simulink model "PC_CONTROL_STATION"  (R2023b)
settings: Solver=FixedStepAuto  StartTime=0.0  StopTime=inf  RelTol=1e-3  EnableMultiTasking=on
InitFcn:
  | if RUN_MODE~=5
  |     % clear rpi;
  |     rpi = raspberrypi(CAR_IP, 'pi', 'LabControl');
  |     stopModel(rpi,'CAR_CONTROL_SYSTEM')
  |     while isModelRunning(rpi,'CAR_CONTROL_SYSTEM')
  |          stopModel(rpi,'CAR_CONTROL_SYSTEM')
  |     end
  |     runModel(rpi,'CAR_CONTROL_SYSTEM')
  |      while isModelRunning(rpi,'CAR_CONTROL_SYSTEM')==false
  |          runModel(rpi,'CAR_CONTROL_SYSTEM')
  |      end
  |      % clear rpi;
  | end
StopFcn:
  | if RUN_MODE~=5
  |    clear rpi;
  |    rpi = raspberrypi(CAR_IP, 'pi', 'LabControl');
  |    stopModel(rpi,'CAR_CONTROL_SYSTEM')
  |    while isModelRunning(rpi,'CAR_CONTROL_SYSTEM')
  |    end
  |    clear rpi;
  | end
model workspace (MAT data in the model file):
  SL_ROS_VariableLengthArrays_MaxSizes : object (value not decoded)
values from neighbouring files (symbols this model uses):
  data = theClient.GetLastFrameOfData()    [FuncMotive.m]
undefined symbols (not defined in the file or in its folder): CONTROL, CONTROL_INI, data_SL_Info, MD25, MSG, SAMPLING_TIME, Standard_Devices, SYSID_INPUT, TCP_Protocol, UDP_Protocol
libraries: simulink x51, sldrtlib x46, dspsigattribs x7, ros2lib x3, ctrlSharedLib x2, aerolibanimutils x1
(part 3 of 8)

== system PC_CONTROL_STATION/HARDWARE/RT_MONITORING/TCP 106/MSG_TX  ==
  Enable : EnablePort
  Data Store Read1 : DataStoreRead  DataStoreName=MSG  SampleTime=CONTROL_INI.PARAM.COMM_SAMPLING_TIME  DataStoreElements=MSG.TX_BUFFER(:,1)  IndexOptions=Index vector (dialog)  Indices=1  OutputSizes=1
  Packet Output : sldrtlib/Packet Output  SampleTime=CONTROL_INI.PARAM.COMM_SAMPLING_TIME  MaxMissedTicks=50  ShowMissedTicks=off  YieldWhenWaiting=off  DrvName=Standard_Devices/TCP_Protocol  DrvAddress=27000  DrvOptions=[0 27001 49 57 50 46 49 54 56 46 48 46 49 48 54 0 0 0 0 0 0 0 0 0 0 0 0 0 0 0 0 0 0 0 0 0 0 0 0 0 0 0 0 0 0 0 0 0 0 0 0 0 0 0 0 0 0 0 0 0 0 0 0 0 0 0 0 0 0 0 0 0 0 0 0 0 0 0 0 0 0 0 0 0 0 0 0 0 0 0 0 0 0 0 0 0 0 0 0 0 0 0 0 0 0 0 0 0 0 0 0 0 0 0 0 0 0 0 0 0 0 0 0 0 0 0 0 0 0 0 0 0 0 0 0 0 0 0 0 0 0 0 0 0 0 0 0 0 0 0 0 0 0 0 0 0 0 0 0 0 0 0 0 0 0 0 0 0 0 0 0 0 0 0 0 0 0 0 0 0 0 0 0 0 0 0 0 0 0 0 0 0 0 0 0 0 0 0 0 0 0 0 0 0 0 0 0 0 0 0 0 0 0 0 0 0 0 0 0 0 0 0 0 0 0 0 0 0 0 0 0 0 0 0 0 0 0 0 0 0 0 0 0 0 0 0 0 0 0 0 0 0 0 0 0 0]  PacketSize=1400  DataTypes={'1400*uint8'}  ShowReady=off  ShowError=off  PacketID=1  ByteOrder=2  InitialValue=[]  FinalValue=[]
      settings: AttributesFormatString=TCP Protocol [27000]
  wires:
  Data Store Read1/1 -> Packet Output/1

== system PC_CONTROL_STATION/HARDWARE/RT_MONITORING/TCP 107/MSG_RX ==
  Bus Assignment : BusAssignment  AssignedSignals=RX_BUFFER
  Data Store Read : DataStoreRead  DataStoreName=MSG  IndexOptions=Index vector (dialog)  Indices=1  OutputSizes=1
  Data Store Write1 : DataStoreWrite  DataStoreName=MSG  IndexOptions=Index vector (dialog)  Indices=1  OutputSizes=1
  Packet Input : sldrtlib/Packet Input  SampleTime=CONTROL_INI.PARAM.COMM_SAMPLING_TIME  MaxMissedTicks=50  ShowMissedTicks=off  YieldWhenWaiting=off  DrvName=Standard_Devices/TCP_Protocol  DrvAddress=27001  DrvOptions=[0 27000 49 57 50 46 49 54 56 46 48 46 49 48 55 0 0 0 0 0 0 0 0 0 0 0 0 0 0 0 0 0 0 0 0 0 0 0 0 0 0 0 0 0 0 0 0 0 0 0 0 0 0 0 0 0 0 0 0 0 0 0 0 0 0 0 0 0 0 0 0 0 0 0 0 0 0 0 0 0 0 0 0 0 0 0 0 0 0 0 0 0 0 0 0 0 0 0 0 0 0 0 0 0 0 0 0 0 0 0 0 0 0 0 0 0 0 0 0 0 0 0 0 0 0 0 0 0 0 0 0 0 0 0 0 0 0 0 0 0 0 0 0 0 0 0 0 0 0 0 0 0 0 0 0 0 0 0 0 0 0 0 0 0 0 0 0 0 0 0 0 0 0 0 0 0 0 0 0 0 0 0 0 0 0 0 0 0 0 0 0 0 0 0 0 0 0 0 0 0 0 0 0 0 0 0 0 0 0 0 0 0 0 0 0 0 0 0 0 0 0 0 0 0 0 0 0 0 0 0 0 0 0 0 0 0 0 0 0 0 0 0 0 0 0 0 0 0 0 0 0 0 0 0 0 0]  PacketSize=1400  DataTypes={'1400*uint8'}  ShowReady=off  ShowError=off  PacketID=1  ByteOrder=2  ShowTimestamp=off
      settings: AttributesFormatString=TCP Protocol [27001]
  wires:
  Bus Assignment/1 -> Data Store Write1/1
  Data Store Read/1 -> Bus Assignment/1
  Packet Input/1 -> Bus Assignment/2

== system PC_CONTROL_STATION/HARDWARE/RT_MONITORING/TCP 107/MSG_TX  ==
  Enable : EnablePort
  Data Store Read1 : DataStoreRead  DataStoreName=MSG  SampleTime=CONTROL_INI.PARAM.COMM_SAMPLING_TIME  DataStoreElements=MSG.TX_BUFFER(:,1)  IndexOptions=Index vector (dialog)  Indices=1  OutputSizes=1
  Packet Output : sldrtlib/Packet Output  SampleTime=CONTROL_INI.PARAM.COMM_SAMPLING_TIME  MaxMissedTicks=50  ShowMissedTicks=off  YieldWhenWaiting=off  DrvName=Standard_Devices/TCP_Protocol  DrvAddress=27000  DrvOptions=[0 27001 49 57 50 46 49 54 56 46 48 46 49 48 55 0 0 0 0 0 0 0 0 0 0 0 0 0 0 0 0 0 0 0 0 0 0 0 0 0 0 0 0 0 0 0 0 0 0 0 0 0 0 0 0 0 0 0 0 0 0 0 0 0 0 0 0 0 0 0 0 0 0 0 0 0 0 0 0 0 0 0 0 0 0 0 0 0 0 0 0 0 0 0 0 0 0 0 0 0 0 0 0 0 0 0 0 0 0 0 0 0 0 0 0 0 0 0 0 0 0 0 0 0 0 0 0 0 0 0 0 0 0 0 0 0 0 0 0 0 0 0 0 0 0 0 0 0 0 0 0 0 0 0 0 0 0 0 0 0 0 0 0 0 0 0 0 0 0 0 0 0 0 0 0 0 0 0 0 0 0 0 0 0 0 0 0 0 0 0 0 0 0 0 0 0 0 0 0 0 0 0 0 0 0 0 0 0 0 0 0 0 0 0 0 0 0 0 0 0 0 0 0 0 0 0 0 0 0 0 0 0 0 0 0 0 0 0 0 0 0 0 0 0 0 0 0 0 0 0 0 0 0 0 0 0]  PacketSize=1400  DataTypes={'1400*uint8'}  ShowReady=off  ShowError=off  PacketID=1  ByteOrder=2  InitialValue=[]  FinalValue=[]
      settings: AttributesFormatString=TCP Protocol [27000]
  wires:
  Data Store Read1/1 -> Packet Output/1

== system PC_CONTROL_STATION/HARDWARE/RT_MONITORING/TCP 108/MSG_RX ==
  Bus Assignment : BusAssignment  AssignedSignals=RX_BUFFER
  Data Store Read : DataStoreRead  DataStoreName=MSG  IndexOptions=Index vector (dialog)  Indices=1  OutputSizes=1
  Data Store Write1 : DataStoreWrite  DataStoreName=MSG  IndexOptions=Index vector (dialog)  Indices=1  OutputSizes=1
  Packet Input : sldrtlib/Packet Input  SampleTime=CONTROL_INI.PARAM.COMM_SAMPLING_TIME  MaxMissedTicks=50  ShowMissedTicks=off  YieldWhenWaiting=off  DrvName=Standard_Devices/TCP_Protocol  DrvAddress=27001  DrvOptions=[0 27000 49 57 50 46 49 54 56 46 48 46 49 48 56 0 0 0 0 0 0 0 0 0 0 0 0 0 0 0 0 0 0 0 0 0 0 0 0 0 0 0 0 0 0 0 0 0 0 0 0 0 0 0 0 0 0 0 0 0 0 0 0 0 0 0 0 0 0 0 0 0 0 0 0 0 0 0 0 0 0 0 0 0 0 0 0 0 0 0 0 0 0 0 0 0 0 0 0 0 0 0 0 0 0 0 0 0 0 0 0 0 0 0 0 0 0 0 0 0 0 0 0 0 0 0 0 0 0 0 0 0 0 0 0 0 0 0 0 0 0 0 0 0 0 0 0 0 0 0 0 0 0 0 0 0 0 0 0 0 0 0 0 0 0 0 0 0 0 0 0 0 0 0 0 0 0 0 0 0 0 0 0 0 0 0 0 0 0 0 0 0 0 0 0 0 0 0 0 0 0 0 0 0 0 0 0 0 0 0 0 0 0 0 0 0 0 0 0 0 0 0 0 0 0 0 0 0 0 0 0 0 0 0 0 0 0 0 0 0 0 0 0 0 0 0 0 0 0 0 0 0 0 0 0 0]  PacketSize=1400  DataTypes={'1400*uint8'}  ShowReady=off  ShowError=off  PacketID=1  ByteOrder=2  ShowTimestamp=off
      settings: AttributesFormatString=TCP Protocol [27001]
  wires:
  Bus Assignment/1 -> Data Store Write1/1
  Data Store Read/1 -> Bus Assignment/1
  Packet Input/1 -> Bus Assignment/2

== system PC_CONTROL_STATION/HARDWARE/RT_MONITORING/TCP 108/MSG_TX  ==
  Enable : EnablePort
  Data Store Read1 : DataStoreRead  DataStoreName=MSG  SampleTime=CONTROL_INI.PARAM.COMM_SAMPLING_TIME  DataStoreElements=MSG.TX_BUFFER(:,1)  IndexOptions=Index vector (dialog)  Indices=1  OutputSizes=1
  Packet Output : sldrtlib/Packet Output  SampleTime=CONTROL_INI.PARAM.COMM_SAMPLING_TIME  MaxMissedTicks=50  ShowMissedTicks=off  YieldWhenWaiting=off  DrvName=Standard_Devices/TCP_Protocol  DrvAddress=27000  DrvOptions=[0 27001 49 57 50 46 49 54 56 46 48 46 49 48 56 0 0 0 0 0 0 0 0 0 0 0 0 0 0 0 0 0 0 0 0 0 0 0 0 0 0 0 0 0 0 0 0 0 0 0 0 0 0 0 0 0 0 0 0 0 0 0 0 0 0 0 0 0 0 0 0 0 0 0 0 0 0 0 0 0 0 0 0 0 0 0 0 0 0 0 0 0 0 0 0 0 0 0 0 0 0 0 0 0 0 0 0 0 0 0 0 0 0 0 0 0 0 0 0 0 0 0 0 0 0 0 0 0 0 0 0 0 0 0 0 0 0 0 0 0 0 0 0 0 0 0 0 0 0 0 0 0 0 0 0 0 0 0 0 0 0 0 0 0 0 0 0 0 0 0 0 0 0 0 0 0 0 0 0 0 0 0 0 0 0 0 0 0 0 0 0 0 0 0 0 0 0 0 0 0 0 0 0 0 0 0 0 0 0 0 0 0 0 0 0 0 0 0 0 0 0 0 0 0 0 0 0 0 0 0 0 0 0 0 0 0 0 0 0 0 0 0 0 0 0 0 0 0 0 0 0 0 0 0 0 0]  PacketSize=1400  DataTypes={'1400*uint8'}  ShowReady=off  ShowError=off  PacketID=1  ByteOrder=2  InitialValue=[]  FinalValue=[]
      settings: AttributesFormatString=TCP Protocol [27000]
  wires:
  Data Store Read1/1 -> Packet Output/1

== system PC_CONTROL_STATION/HARDWARE/RT_MONITORING/TCP 109/MSG_RX ==
  Bus Assignment : BusAssignment  AssignedSignals=RX_BUFFER
  Data Store Read : DataStoreRead  DataStoreName=MSG  IndexOptions=Index vector (dialog)  Indices=1  OutputSizes=1
  Data Store Write1 : DataStoreWrite  DataStoreName=MSG  IndexOptions=Index vector (dialog)  Indices=1  OutputSizes=1
  Packet Input : sldrtlib/Packet Input  SampleTime=CONTROL_INI.PARAM.COMM_SAMPLING_TIME  MaxMissedTicks=50  ShowMissedTicks=off  YieldWhenWaiting=off  DrvName=Standard_Devices/TCP_Protocol  DrvAddress=27001  DrvOptions=[0 27000 49 57 50 46 49 54 56 46 48 46 49 48 57 0 0 0 0 0 0 0 0 0 0 0 0 0 0 0 0 0 0 0 0 0 0 0 0 0 0 0 0 0 0 0 0 0 0 0 0 0 0 0 0 0 0 0 0 0 0 0 0 0 0 0 0 0 0 0 0 0 0 0 0 0 0 0 0 0 0 0 0 0 0 0 0 0 0 0 0 0 0 0 0 0 0 0 0 0 0 0 0 0 0 0 0 0 0 0 0 0 0 0 0 0 0 0 0 0 0 0 0 0 0 0 0 0 0 0 0 0 0 0 0 0 0 0 0 0 0 0 0 0 0 0 0 0 0 0 0 0 0 0 0 0 0 0 0 0 0 0 0 0 0 0 0 0 0 0 0 0 0 0 0 0 0 0 0 0 0 0 0 0 0 0 0 0 0 0 0 0 0 0 0 0 0 0 0 0 0 0 0 0 0 0 0 0 0 0 0 0 0 0 0 0 0 0 0 0 0 0 0 0 0 0 0 0 0 0 0 0 0 0 0 0 0 0 0 0 0 0 0 0 0 0 0 0 0 0 0 0 0 0 0 0]  PacketSize=1400  DataTypes={'1400*uint8'}  ShowReady=off  ShowError=off  PacketID=1  ByteOrder=2  ShowTimestamp=off
      settings: AttributesFormatString=TCP Protocol [27001]
  wires:
  Bus Assignment/1 -> Data Store Write1/1
  Data Store Read/1 -> Bus Assignment/1
  Packet Input/1 -> Bus Assignment/2

== system PC_CONTROL_STATION/HARDWARE/RT_MONITORING/TCP 109/MSG_TX  ==
  Enable : EnablePort
  Data Store Read1 : DataStoreRead  DataStoreName=MSG  SampleTime=CONTROL_INI.PARAM.COMM_SAMPLING_TIME  DataStoreElements=MSG.TX_BUFFER(:,1)  IndexOptions=Index vector (dialog)  Indices=1  OutputSizes=1
  Packet Output : sldrtlib/Packet Output  SampleTime=CONTROL_INI.PARAM.COMM_SAMPLING_TIME  MaxMissedTicks=50  ShowMissedTicks=off  YieldWhenWaiting=off  DrvName=Standard_Devices/TCP_Protocol  DrvAddress=27000  DrvOptions=[0 27001 49 57 50 46 49 54 56 46 48 46 49 48 57 0 0 0 0 0 0 0 0 0 0 0 0 0 0 0 0 0 0 0 0 0 0 0 0 0 0 0 0 0 0 0 0 0 0 0 0 0 0 0 0 0 0 0 0 0 0 0 0 0 0 0 0 0 0 0 0 0 0 0 0 0 0 0 0 0 0 0 0 0 0 0 0 0 0 0 0 0 0 0 0 0 0 0 0 0 0 0 0 0 0 0 0 0 0 0 0 0 0 0 0 0 0 0 0 0 0 0 0 0 0 0 0 0 0 0 0 0 0 0 0 0 0 0 0 0 0 0 0 0 0 0 0 0 0 0 0 0 0 0 0 0 0 0 0 0 0 0 0 0 0 0 0 0 0 0 0 0 0 0 0 0 0 0 0 0 0 0 0 0 0 0 0 0 0 0 0 0 0 0 0 0 0 0 0 0 0 0 0 0 0 0 0 0 0 0 0 0 0 0 0 0 0 0 0 0 0 0 0 0 0 0 0 0 0 0 0 0 0 0 0 0 0 0 0 0 0 0 0 0 0 0 0 0 0 0 0 0 0 0 0 0]  PacketSize=1400  DataTypes={'1400*uint8'}  ShowReady=off  ShowError=off  PacketID=1  ByteOrder=2  InitialValue=[]  FinalValue=[]
      settings: AttributesFormatString=TCP Protocol [27000]
  wires:
  Data Store Read1/1 -> Packet Output/1

== system PC_CONTROL_STATION/HARDWARE/RT_MONITORING/TCP 110/MSG_RX ==
  Bus Assignment : BusAssignment  AssignedSignals=RX_BUFFER
  Data Store Read : DataStoreRead  DataStoreName=MSG  IndexOptions=Index vector (dialog)  Indices=1  OutputSizes=1
  Data Store Write1 : DataStoreWrite  DataStoreName=MSG  IndexOptions=Index vector (dialog)  Indices=1  OutputSizes=1
  Packet Input : sldrtlib/Packet Input  SampleTime=CONTROL_INI.PARAM.COMM_SAMPLING_TIME  MaxMissedTicks=50  ShowMissedTicks=off  YieldWhenWaiting=off  DrvName=Standard_Devices/TCP_Protocol  DrvAddress=27001  DrvOptions=[0 27000 49 57 50 46 49 54 56 46 48 46 49 49 48 0 0 0 0 0 0 0 0 0 0 0 0 0 0 0 0 0 0 0 0 0 0 0 0 0 0 0 0 0 0 0 0 0 0 0 0 0 0 0 0 0 0 0 0 0 0 0 0 0 0 0 0 0 0 0 0 0 0 0 0 0 0 0 0 0 0 0 0 0 0 0 0 0 0 0 0 0 0 0 0 0 0 0 0 0 0 0 0 0 0 0 0 0 0 0 0 0 0 0 0 0 0 0 0 0 0 0 0 0 0 0 0 0 0 0 0 0 0 0 0 0 0 0 0 0 0 0 0 0 0 0 0 0 0 0 0 0 0 0 0 0 0 0 0 0 0 0 0 0 0 0 0 0 0 0 0 0 0 0 0 0 0 0 0 0 0 0 0 0 0 0 0 0 0 0 0 0 0 0 0 0 0 0 0 0 0 0 0 0 0 0 0 0 0 0 0 0 0 0 0 0 0 0 0 0 0 0 0 0 0 0 0 0 0 0 0 0 0 0 0 0 0 0 0 0 0 0 0 0 0 0 0 0 0 0 0 0 0 0 0 0]  PacketSize=1400  DataTypes={'1400*uint8'}  ShowReady=off  ShowError=off  PacketID=1  ByteOrder=2  ShowTimestamp=off
      settings: AttributesFormatString=TCP Protocol [27001]
  wires:
  Bus Assignment/1 -> Data Store Write1/1
  Data Store Read/1 -> Bus Assignment/1
  Packet Input/1 -> Bus Assignment/2

== system PC_CONTROL_STATION/HARDWARE/RT_MONITORING/TCP 110/MSG_TX  ==
  Enable : EnablePort
  Data Store Read1 : DataStoreRead  DataStoreName=MSG  SampleTime=CONTROL_INI.PARAM.COMM_SAMPLING_TIME  DataStoreElements=MSG.TX_BUFFER(:,1)  IndexOptions=Index vector (dialog)  Indices=1  OutputSizes=1
  Packet Output : sldrtlib/Packet Output  SampleTime=CONTROL_INI.PARAM.COMM_SAMPLING_TIME  MaxMissedTicks=50  ShowMissedTicks=off  YieldWhenWaiting=off  DrvName=Standard_Devices/TCP_Protocol  DrvAddress=27000  DrvOptions=[0 27001 49 57 50 46 49 54 56 46 48 46 49 49 48 0 0 0 0 0 0 0 0 0 0 0 0 0 0 0 0 0 0 0 0 0 0 0 0 0 0 0 0 0 0 0 0 0 0 0 0 0 0 0 0 0 0 0 0 0 0 0 0 0 0 0 0 0 0 0 0 0 0 0 0 0 0 0 0 0 0 0 0 0 0 0 0 0 0 0 0 0 0 0 0 0 0 0 0 0 0 0 0 0 0 0 0 0 0 0 0 0 0 0 0 0 0 0 0 0 0 0 0 0 0 0 0 0 0 0 0 0 0 0 0 0 0 0 0 0 0 0 0 0 0 0 0 0 0 0 0 0 0 0 0 0 0 0 0 0 0 0 0 0 0 0 0 0 0 0 0 0 0 0 0 0 0 0 0 0 0 0 0 0 0 0 0 0 0 0 0 0 0 0 0 0 0 0 0 0 0 0 0 0 0 0 0 0 0 0 0 0 0 0 0 0 0 0 0 0 0 0 0 0 0 0 0 0 0 0 0 0 0 0 0 0 0 0 0 0 0 0 0 0 0 0 0 0 0 0 0 0 0 0 0 0]  PacketSize=1400  DataTypes={'1400*uint8'}  ShowReady=off  ShowError=off  PacketID=1  ByteOrder=2  InitialValue=[]  FinalValue=[]
      settings: AttributesFormatString=TCP Protocol [27000]
  wires:
  Data Store Read1/1 -> Packet Output/1

== system PC_CONTROL_STATION/HARDWARE/RT_MONITORING/TCP 111/MSG_RX ==
  Bus Assignment : BusAssignment  AssignedSignals=RX_BUFFER
  Data Store Read : DataStoreRead  DataStoreName=MSG  IndexOptions=Index vector (dialog)  Indices=1  OutputSizes=1
  Data Store Write1 : DataStoreWrite  DataStoreName=MSG  IndexOptions=Index vector (dialog)  Indices=1  OutputSizes=1
  Packet Input : sldrtlib/Packet Input  SampleTime=CONTROL_INI.PARAM.COMM_SAMPLING_TIME  MaxMissedTicks=50  ShowMissedTicks=off  YieldWhenWaiting=off  DrvName=Standard_Devices/TCP_Protocol  DrvAddress=27001  DrvOptions=[0 27000 49 57 50 46 49 54 56 46 48 46 49 49 49 0 0 0 0 0 0 0 0 0 0 0 0 0 0 0 0 0 0 0 0 0 0 0 0 0 0 0 0 0 0 0 0 0 0 0 0 0 0 0 0 0 0 0 0 0 0 0 0 0 0 0 0 0 0 0 0 0 0 0 0 0 0 0 0 0 0 0 0 0 0 0 0 0 0 0 0 0 0 0 0 0 0 0 0 0 0 0 0 0 0 0 0 0 0 0 0 0 0 0 0 0 0 0 0 0 0 0 0 0 0 0 0 0 0 0 0 0 0 0 0 0 0 0 0 0 0 0 0 0 0 0 0 0 0 0 0 0 0 0 0 0 0 0 0 0 0 0 0 0 0 0 0 0 0 0 0 0 0 0 0 0 0 0 0 0 0 0 0 0 0 0 0 0 0 0 0 0 0 0 0 0 0 0 0 0 0 0 0 0 0 0 0 0 0 0 0 0 0 0 0 0 0 0 0 0 0 0 0 0 0 0 0 0 0 0 0 0 0 0 0 0 0 0 0 0 0 0 0 0 0 0 0 0 0 0 0 0 0 0 0 0]  PacketSize=1400  DataTypes={'1400*uint8'}  ShowReady=off  ShowError=off  PacketID=1  ByteOrder=2  ShowTimestamp=off
      settings: AttributesFormatString=TCP Protocol [27001]
  wires:
  Bus Assignment/1 -> Data Store Write1/1
  Data Store Read/1 -> Bus Assignment/1
  Packet Input/1 -> Bus Assignment/2

== system PC_CONTROL_STATION/HARDWARE/RT_MONITORING/TCP 111/MSG_TX  ==
  Enable : EnablePort
  Data Store Read1 : DataStoreRead  DataStoreName=MSG  SampleTime=CONTROL_INI.PARAM.COMM_SAMPLING_TIME  DataStoreElements=MSG.TX_BUFFER(:,1)  IndexOptions=Index vector (dialog)  Indices=1  OutputSizes=1
  Packet Output : sldrtlib/Packet Output  SampleTime=CONTROL_INI.PARAM.COMM_SAMPLING_TIME  MaxMissedTicks=50  ShowMissedTicks=off  YieldWhenWaiting=off  DrvName=Standard_Devices/TCP_Protocol  DrvAddress=27000  DrvOptions=[0 27001 49 57 50 46 49 54 56 46 48 46 49 49 49 0 0 0 0 0 0 0 0 0 0 0 0 0 0 0 0 0 0 0 0 0 0 0 0 0 0 0 0 0 0 0 0 0 0 0 0 0 0 0 0 0 0 0 0 0 0 0 0 0 0 0 0 0 0 0 0 0 0 0 0 0 0 0 0 0 0 0 0 0 0 0 0 0 0 0 0 0 0 0 0 0 0 0 0 0 0 0 0 0 0 0 0 0 0 0 0 0 0 0 0 0 0 0 0 0 0 0 0 0 0 0 0 0 0 0 0 0 0 0 0 0 0 0 0 0 0 0 0 0 0 0 0 0 0 0 0 0 0 0 0 0 0 0 0 0 0 0 0 0 0 0 0 0 0 0 0 0 0 0 0 0 0 0 0 0 0 0 0 0 0 0 0 0 0 0 0 0 0 0 0 0 0 0 0 0 0 0 0 0 0 0 0 0 0 0 0 0 0 0 0 0 0 0 0 0 0 0 0 0 0 0 0 0 0 0 0 0 0 0 0 0 0 0 0 0 0 0 0 0 0 0 0 0 0 0 0 0 0 0 0 0]  PacketSize=1400  DataTypes={'1400*uint8'}  ShowReady=off  ShowError=off  PacketID=1  ByteOrder=2  InitialValue=[]  FinalValue=[]
      settings: AttributesFormatString=TCP Protocol [27000]
  wires:
  Data Store Read1/1 -> Packet Output/1

== system PC_CONTROL_STATION/HARDWARE/RT_MONITORING/TCP 112/MSG_RX ==
  Bus Assignment : BusAssignment  AssignedSignals=RX_BUFFER
  Data Store Read : DataStoreRead  DataStoreName=MSG  IndexOptions=Index vector (dialog)  Indices=1  OutputSizes=1
  Data Store Write1 : DataStoreWrite  DataStoreName=MSG  IndexOptions=Index vector (dialog)  Indices=1  OutputSizes=1
  Packet Input : sldrtlib/Packet Input  SampleTime=CONTROL_INI.PARAM.COMM_SAMPLING_TIME  MaxMissedTicks=50  ShowMissedTicks=off  YieldWhenWaiting=off  DrvName=Standard_Devices/TCP_Protocol  DrvAddress=27001  DrvOptions=[0 27000 49 57 50 46 49 54 56 46 48 46 49 49 50 0 0 0 0 0 0 0 0 0 0 0 0 0 0 0 0 0 0 0 0 0 0 0 0 0 0 0 0 0 0 0 0 0 0 0 0 0 0 0 0 0 0 0 0 0 0 0 0 0 0 0 0 0 0 0 0 0 0 0 0 0 0 0 0 0 0 0 0 0 0 0 0 0 0 0 0 0 0 0 0 0 0 0 0 0 0 0 0 0 0 0 0 0 0 0 0 0 0 0 0 0 0 0 0 0 0 0 0 0 0 0 0 0 0 0 0 0 0 0 0 0 0 0 0 0 0 0 0 0 0 0 0 0 0 0 0 0 0 0 0 0 0 0 0 0 0 0 0 0 0 0 0 0 0 0 0 0 0 0 0 0 0 0 0 0 0 0 0 0 0 0 0 0 0 0 0 0 0 0 0 0 0 0 0 0 0 0 0 0 0 0 0 0 0 0 0 0 0 0 0 0 0 0 0 0 0 0 0 0 0 0 0 0 0 0 0 0 0 0 0 0 0 0 0 0 0 0 0 0 0 0 0 0 0 0 0 0 0 0 0 0]  PacketSize=1400  DataTypes={'1400*uint8'}  ShowReady=off  ShowError=off  PacketID=1  ByteOrder=2  ShowTimestamp=off
      settings: AttributesFormatString=TCP Protocol [27001]
  wires:
  Bus Assignment/1 -> Data Store Write1/1
  Data Store Read/1 -> Bus Assignment/1
  Packet Input/1 -> Bus Assignment/2

== system PC_CONTROL_STATION/HARDWARE/RT_MONITORING/TCP 112/MSG_TX  ==
  Enable : EnablePort
  Data Store Read1 : DataStoreRead  DataStoreName=MSG  SampleTime=CONTROL_INI.PARAM.COMM_SAMPLING_TIME  DataStoreElements=MSG.TX_BUFFER(:,1)  IndexOptions=Index vector (dialog)  Indices=1  OutputSizes=1
  Packet Output : sldrtlib/Packet Output  SampleTime=CONTROL_INI.PARAM.COMM_SAMPLING_TIME  MaxMissedTicks=50  ShowMissedTicks=off  YieldWhenWaiting=off  DrvName=Standard_Devices/TCP_Protocol  DrvAddress=27000  DrvOptions=[0 27001 49 57 50 46 49 54 56 46 48 46 49 49 50 0 0 0 0 0 0 0 0 0 0 0 0 0 0 0 0 0 0 0 0 0 0 0 0 0 0 0 0 0 0 0 0 0 0 0 0 0 0 0 0 0 0 0 0 0 0 0 0 0 0 0 0 0 0 0 0 0 0 0 0 0 0 0 0 0 0 0 0 0 0 0 0 0 0 0 0 0 0 0 0 0 0 0 0 0 0 0 0 0 0 0 0 0 0 0 0 0 0 0 0 0 0 0 0 0 0 0 0 0 0 0 0 0 0 0 0 0 0 0 0 0 0 0 0 0 0 0 0 0 0 0 0 0 0 0 0 0 0 0 0 0 0 0 0 0 0 0 0 0 0 0 0 0 0 0 0 0 0 0 0 0 0 0 0 0 0 0 0 0 0 0 0 0 0 0 0 0 0 0 0 0 0 0 0 0 0 0 0 0 0 0 0 0 0 0 0 0 0 0 0 0 0 0 0 0 0 0 0 0 0 0 0 0 0 0 0 0 0 0 0 0 0 0 0 0 0 0 0 0 0 0 0 0 0 0 0 0 0 0 0 0]  PacketSize=1400  DataTypes={'1400*uint8'}  ShowReady=off  ShowError=off  PacketID=1  ByteOrder=2  InitialValue=[]  FinalValue=[]
      settings: AttributesFormatString=TCP Protocol [27000]
  wires:
  Data Store Read1/1 -> Packet Output/1

== system PC_CONTROL_STATION/HARDWARE/RT_MONITORING/TCP 113/MSG_RX ==
  Bus Assignment : BusAssignment  AssignedSignals=RX_BUFFER
  Data Store Read : DataStoreRead  DataStoreName=MSG  IndexOptions=Index vector (dialog)  Indices=1  OutputSizes=1
  Data Store Write1 : DataStoreWrite  DataStoreName=MSG  IndexOptions=Index vector (dialog)  Indices=1  OutputSizes=1
  Packet Input : sldrtlib/Packet Input  SampleTime=CONTROL_INI.PARAM.COMM_SAMPLING_TIME  MaxMissedTicks=50  ShowMissedTicks=off  YieldWhenWaiting=off  DrvName=Standard_Devices/TCP_Protocol  DrvAddress=27001  DrvOptions=[0 27000 49 57 50 46 49 54 56 46 48 46 49 49 51 0 0 0 0 0 0 0 0 0 0 0 0 0 0 0 0 0 0 0 0 0 0 0 0 0 0 0 0 0 0 0 0 0 0 0 0 0 0 0 0 0 0 0 0 0 0 0 0 0 0 0 0 0 0 0 0 0 0 0 0 0 0 0 0 0 0 0 0 0 0 0 0 0 0 0 0 0 0 0 0 0 0 0 0 0 0 0 0 0 0 0 0 0 0 0 0 0 0 0 0 0 0 0 0 0 0 0 0 0 0 0 0 0 0 0 0 0 0 0 0 0 0 0 0 0 0 0 0 0 0 0 0 0 0 0 0 0 0 0 0 0 0 0 0 0 0 0 0 0 0 0 0 0 0 0 0 0 0 0 0 0 0 0 0 0 0 0 0 0 0 0 0 0 0 0 0 0 0 0 0 0 0 0 0 0 0 0 0 0 0 0 0 0 0 0 0 0 0 0 0 0 0 0 0 0 0 0 0 0 0 0 0 0 0 0 0 0 0 0 0 0 0 0 0 0 0 0 0 0 0 0 0 0 0 0 0 0 0 0 0 0]  PacketSize=1400  DataTypes={'1400*uint8'}  ShowReady=off  ShowError=off  PacketID=1  ByteOrder=2  ShowTimestamp=off
      settings: AttributesFormatString=TCP Protocol [27001]
  wires:
  Bus Assignment/1 -> Data Store Write1/1
  Data Store Read/1 -> Bus Assignment/1
  Packet Input/1 -> Bus Assignment/2

== system PC_CONTROL_STATION/HARDWARE/RT_MONITORING/TCP 113/MSG_TX  ==
  Enable : EnablePort
  Data Store Read1 : DataStoreRead  DataStoreName=MSG  SampleTime=CONTROL_INI.PARAM.COMM_SAMPLING_TIME  DataStoreElements=MSG.TX_BUFFER(:,1)  IndexOptions=Index vector (dialog)  Indices=1  OutputSizes=1
  Packet Output : sldrtlib/Packet Output  SampleTime=CONTROL_INI.PARAM.COMM_SAMPLING_TIME  MaxMissedTicks=50  ShowMissedTicks=off  YieldWhenWaiting=off  DrvName=Standard_Devices/TCP_Protocol  DrvAddress=27000  DrvOptions=[0 27001 49 57 50 46 49 54 56 46 48 46 49 49 51 0 0 0 0 0 0 0 0 0 0 0 0 0 0 0 0 0 0 0 0 0 0 0 0 0 0 0 0 0 0 0 0 0 0 0 0 0 0 0 0 0 0 0 0 0 0 0 0 0 0 0 0 0 0 0 0 0 0 0 0 0 0 0 0 0 0 0 0 0 0 0 0 0 0 0 0 0 0 0 0 0 0 0 0 0 0 0 0 0 0 0 0 0 0 0 0 0 0 0 0 0 0 0 0 0 0 0 0 0 0 0 0 0 0 0 0 0 0 0 0 0 0 0 0 0 0 0 0 0 0 0 0 0 0 0 0 0 0 0 0 0 0 0 0 0 0 0 0 0 0 0 0 0 0 0 0 0 0 0 0 0 0 0 0 0 0 0 0 0 0 0 0 0 0 0 0 0 0 0 0 0 0 0 0 0 0 0 0 0 0 0 0 0 0 0 0 0 0 0 0 0 0 0 0 0 0 0 0 0 0 0 0 0 0 0 0 0 0 0 0 0 0 0 0 0 0 0 0 0 0 0 0 0 0 0 0 0 0 0 0 0]  PacketSize=1400  DataTypes={'1400*uint8'}  ShowReady=off  ShowError=off  PacketID=1  ByteOrder=2  InitialValue=[]  FinalValue=[]
      settings: AttributesFormatString=TCP Protocol [27000]
  wires:
  Data Store Read1/1 -> Packet Output/1

== system PC_CONTROL_STATION/HARDWARE/RT_MONITORING/TCP 114/MSG_RX ==
  Bus Assignment : BusAssignment  AssignedSignals=RX_BUFFER
  Data Store Read : DataStoreRead  DataStoreName=MSG  IndexOptions=Index vector (dialog)  Indices=1  OutputSizes=1
  Data Store Write1 : DataStoreWrite  DataStoreName=MSG  IndexOptions=Index vector (dialog)  Indices=1  OutputSizes=1
  Packet Input : sldrtlib/Packet Input  SampleTime=CONTROL_INI.PARAM.COMM_SAMPLING_TIME  MaxMissedTicks=50  ShowMissedTicks=off  YieldWhenWaiting=off  DrvName=Standard_Devices/TCP_Protocol  DrvAddress=27001  DrvOptions=[0 27000 49 57 50 46 49 54 56 46 49 46 49 50 0 0 0 0 0 0 0 0 0 0 0 0 0 0 0 0 0 0 0 0 0 0 0 0 0 0 0 0 0 0 0 0 0 0 0 0 0 0 0 0 0 0 0 0 0 0 0 0 0 0 0 0 0 0 0 0 0 0 0 0 0 0 0 0 0 0 0 0 0 0 0 0 0 0 0 0 0 0 0 0 0 0 0 0 0 0 0 0 0 0 0 0 0 0 0 0 0 0 0 0 0 0 0 0 0 0 0 0 0 0 0 0 0 0 0 0 0 0 0 0 0 0 0 0 0 0 0 0 0 0 0 0 0 0 0 0 0 0 0 0 0 0 0 0 0 0 0 0 0 0 0 0 0 0 0 0 0 0 0 0 0 0 0 0 0 0 0 0 0 0 0 0 0 0 0 0 0 0 0 0 0 0 0 0 0 0 0 0 0 0 0 0 0 0 0 0 0 0 0 0 0 0 0 0 0 0 0 0 0 0 0 0 0 0 0 0 0 0 0 0 0 0 0 0 0 0 0 0 0 0 0 0 0 0 0 0 0 0 0 0 0 0]  PacketSize=1400  DataTypes={'1400*uint8'}  ShowReady=off  ShowError=off  PacketID=1  ByteOrder=2  ShowTimestamp=off
      settings: AttributesFormatString=TCP Protocol [27001]
  wires:
  Bus Assignment/1 -> Data Store Write1/1
  Data Store Read/1 -> Bus Assignment/1
  Packet Input/1 -> Bus Assignment/2

== system PC_CONTROL_STATION/HARDWARE/RT_MONITORING/TCP 114/MSG_TX  ==
  Enable : EnablePort
  Data Store Read1 : DataStoreRead  DataStoreName=MSG  SampleTime=CONTROL_INI.PARAM.COMM_SAMPLING_TIME  DataStoreElements=MSG.TX_BUFFER(:,1)  IndexOptions=Index vector (dialog)  Indices=1  OutputSizes=1
  Packet Output : sldrtlib/Packet Output  SampleTime=CONTROL_INI.PARAM.COMM_SAMPLING_TIME  MaxMissedTicks=50  ShowMissedTicks=off  YieldWhenWaiting=off  DrvName=Standard_Devices/TCP_Protocol  DrvAddress=27000  DrvOptions=[0 27001 49 57 50 46 49 54 56 46 49 46 49 50 0 0 0 0 0 0 0 0 0 0 0 0 0 0 0 0 0 0 0 0 0 0 0 0 0 0 0 0 0 0 0 0 0 0 0 0 0 0 0 0 0 0 0 0 0 0 0 0 0 0 0 0 0 0 0 0 0 0 0 0 0 0 0 0 0 0 0 0 0 0 0 0 0 0 0 0 0 0 0 0 0 0 0 0 0 0 0 0 0 0 0 0 0 0 0 0 0 0 0 0 0 0 0 0 0 0 0 0 0 0 0 0 0 0 0 0 0 0 0 0 0 0 0 0 0 0 0 0 0 0 0 0 0 0 0 0 0 0 0 0 0 0 0 0 0 0 0 0 0 0 0 0 0 0 0 0 0 0 0 0 0 0 0 0 0 0 0 0 0 0 0 0 0 0 0 0 0 0 0 0 0 0 0 0 0 0 0 0 0 0 0 0 0 0 0 0 0 0 0 0 0 0 0 0 0 0 0 0 0 0 0 0 0 0 0 0 0 0 0 0 0 0 0 0 0 0 0 0 0 0 0 0 0 0 0 0 0 0 0 0 0 0]  PacketSize=1400  DataTypes={'1400*uint8'}  ShowReady=off  ShowError=off  PacketID=1  ByteOrder=2  InitialValue=[]  FinalValue=[]
      settings: AttributesFormatString=TCP Protocol [27000]
  wires:
  Data Store Read1/1 -> Packet Output/1

== system PC_CONTROL_STATION/HARDWARE/RT_MONITORING/TCP 115/MSG_RX ==
  Bus Assignment : BusAssignment  AssignedSignals=RX_BUFFER
  Data Store Read : DataStoreRead  DataStoreName=MSG  IndexOptions=Index vector (dialog)  Indices=1  OutputSizes=1
  Data Store Write1 : DataStoreWrite  DataStoreName=MSG  IndexOptions=Index vector (dialog)  Indices=1  OutputSizes=1
  Packet Input : sldrtlib/Packet Input  SampleTime=CONTROL_INI.PARAM.COMM_SAMPLING_TIME  MaxMissedTicks=50  ShowMissedTicks=off  YieldWhenWaiting=off  DrvName=Standard_Devices/TCP_Protocol  DrvAddress=27001  DrvOptions=[0 27000 49 57 50 46 49 54 56 46 48 46 49 49 53 0 0 0 0 0 0 0 0 0 0 0 0 0 0 0 0 0 0 0 0 0 0 0 0 0 0 0 0 0 0 0 0 0 0 0 0 0 0 0 0 0 0 0 0 0 0 0 0 0 0 0 0 0 0 0 0 0 0 0 0 0 0 0 0 0 0 0 0 0 0 0 0 0 0 0 0 0 0 0 0 0 0 0 0 0 0 0 0 0 0 0 0 0 0 0 0 0 0 0 0 0 0 0 0 0 0 0 0 0 0 0 0 0 0 0 0 0 0 0 0 0 0 0 0 0 0 0 0 0 0 0 0 0 0 0 0 0 0 0 0 0 0 0 0 0 0 0 0 0 0 0 0 0 0 0 0 0 0 0 0 0 0 0 0 0 0 0 0 0 0 0 0 0 0 0 0 0 0 0 0 0 0 0 0 0 0 0 0 0 0 0 0 0 0 0 0 0 0 0 0 0 0 0 0 0 0 0 0 0 0 0 0 0 0 0 0 0 0 0 0 0 0 0 0 0 0 0 0 0 0 0 0 0 0 0 0 0 0 0 0 0]  PacketSize=1400  DataTypes={'1400*uint8'}  ShowReady=off  ShowError=off  PacketID=1  ByteOrder=2  ShowTimestamp=off
      settings: AttributesFormatString=TCP Protocol [27001]
  wires:
  Bus Assignment/1 -> Data Store Write1/1
  Data Store Read/1 -> Bus Assignment/1
  Packet Input/1 -> Bus Assignment/2

== system PC_CONTROL_STATION/HARDWARE/RT_MONITORING/TCP 115/MSG_TX  ==
  Enable : EnablePort
  Data Store Read1 : DataStoreRead  DataStoreName=MSG  SampleTime=CONTROL_INI.PARAM.COMM_SAMPLING_TIME  DataStoreElements=MSG.TX_BUFFER(:,1)  IndexOptions=Index vector (dialog)  Indices=1  OutputSizes=1
  Packet Output : sldrtlib/Packet Output  SampleTime=CONTROL_INI.PARAM.COMM_SAMPLING_TIME  MaxMissedTicks=50  ShowMissedTicks=off  YieldWhenWaiting=off  DrvName=Standard_Devices/TCP_Protocol  DrvAddress=27000  DrvOptions=[0 27001 49 57 50 46 49 54 56 46 48 46 49 49 53 0 0 0 0 0 0 0 0 0 0 0 0 0 0 0 0 0 0 0 0 0 0 0 0 0 0 0 0 0 0 0 0 0 0 0 0 0 0 0 0 0 0 0 0 0 0 0 0 0 0 0 0 0 0 0 0 0 0 0 0 0 0 0 0 0 0 0 0 0 0 0 0 0 0 0 0 0 0 0 0 0 0 0 0 0 0 0 0 0 0 0 0 0 0 0 0 0 0 0 0 0 0 0 0 0 0 0 0 0 0 0 0 0 0 0 0 0 0 0 0 0 0 0 0 0 0 0 0 0 0 0 0 0 0 0 0 0 0 0 0 0 0 0 0 0 0 0 0 0 0 0 0 0 0 0 0 0 0 0 0 0 0 0 0 0 0 0 0 0 0 0 0 0 0 0 0 0 0 0 0 0 0 0 0 0 0 0 0 0 0 0 0 0 0 0 0 0 0 0 0 0 0 0 0 0 0 0 0 0 0 0 0 0 0 0 0 0 0 0 0 0 0 0 0 0 0 0 0 0 0 0 0 0 0 0 0 0 0 0 0 0]  PacketSize=1400  DataTypes={'1400*uint8'}  ShowReady=off  ShowError=off  PacketID=1  ByteOrder=2  InitialValue=[]  FinalValue=[]
      settings: AttributesFormatString=TCP Protocol [27000]
  wires:
  Data Store Read1/1 -> Packet Output/1

== system PC_CONTROL_STATION/HARDWARE/RT_MONITORING/TCP 116/MSG_RX ==
  Bus Assignment : BusAssignment  AssignedSignals=RX_BUFFER
  Data Store Read : DataStoreRead  DataStoreName=MSG  IndexOptions=Index vector (dialog)  Indices=1  OutputSizes=1
  Data Store Write1 : DataStoreWrite  DataStoreName=MSG  IndexOptions=Index vector (dialog)  Indices=1  OutputSizes=1
  Packet Input : sldrtlib/Packet Input  SampleTime=CONTROL_INI.PARAM.COMM_SAMPLING_TIME  MaxMissedTicks=50  ShowMissedTicks=off  YieldWhenWaiting=off  DrvName=Standard_Devices/TCP_Protocol  DrvAddress=27001  DrvOptions=[0 27000 49 57 50 46 49 54 56 46 48 46 49 49 54 0 0 0 0 0 0 0 0 0 0 0 0 0 0 0 0 0 0 0 0 0 0 0 0 0 0 0 0 0 0 0 0 0 0 0 0 0 0 0 0 0 0 0 0 0 0 0 0 0 0 0 0 0 0 0 0 0 0 0 0 0 0 0 0 0 0 0 0 0 0 0 0 0 0 0 0 0 0 0 0 0 0 0 0 0 0 0 0 0 0 0 0 0 0 0 0 0 0 0 0 0 0 0 0 0 0 0 0 0 0 0 0 0 0 0 0 0 0 0 0 0 0 0 0 0 0 0 0 0 0 0 0 0 0 0 0 0 0 0 0 0 0 0 0 0 0 0 0 0 0 0 0 0 0 0 0 0 0 0 0 0 0 0 0 0 0 0 0 0 0 0 0 0 0 0 0 0 0 0 0 0 0 0 0 0 0 0 0 0 0 0 0 0 0 0 0 0 0 0 0 0 0 0 0 0 0 0 0 0 0 0 0 0 0 0 0 0 0 0 0 0 0 0 0 0 0 0 0 0 0 0 0 0 0 0 0 0 0 0 0 0]  PacketSize=500  DataTypes={'500*uint8'}  ShowReady=off  ShowError=off  PacketID=1  ByteOrder=2  ShowTimestamp=off
      settings: AttributesFormatString=TCP Protocol [27001]
  wires:
  Bus Assignment/1 -> Data Store Write1/1
  Data Store Read/1 -> Bus Assignment/1
  Packet Input/1 -> Bus Assignment/2

== system PC_CONTROL_STATION/HARDWARE/RT_MONITORING/TCP 116/MSG_TX  ==
  Enable : EnablePort
  Data Store Read1 : DataStoreRead  DataStoreName=MSG  SampleTime=CONTROL_INI.PARAM.COMM_SAMPLING_TIME  DataStoreElements=MSG.TX_BUFFER(:,1)  IndexOptions=Index vector (dialog)  Indices=1  OutputSizes=1
  Packet Output : sldrtlib/Packet Output  SampleTime=CONTROL_INI.PARAM.COMM_SAMPLING_TIME  MaxMissedTicks=50  ShowMissedTicks=off  YieldWhenWaiting=off  DrvName=Standard_Devices/TCP_Protocol  DrvAddress=27000  DrvOptions=[0 27001 49 57 50 46 49 54 56 46 48 46 49 49 54 0 0 0 0 0 0 0 0 0 0 0 0 0 0 0 0 0 0 0 0 0 0 0 0 0 0 0 0 0 0 0 0 0 0 0 0 0 0 0 0 0 0 0 0 0 0 0 0 0 0 0 0 0 0 0 0 0 0 0 0 0 0 0 0 0 0 0 0 0 0 0 0 0 0 0 0 0 0 0 0 0 0 0 0 0 0 0 0 0 0 0 0 0 0 0 0 0 0 0 0 0 0 0 0 0 0 0 0 0 0 0 0 0 0 0 0 0 0 0 0 0 0 0 0 0 0 0 0 0 0 0 0 0 0 0 0 0 0 0 0 0 0 0 0 0 0 0 0 0 0 0 0 0 0 0 0 0 0 0 0 0 0 0 0 0 0 0 0 0 0 0 0 0 0 0 0 0 0 0 0 0 0 0 0 0 0 0 0 0 0 0 0 0 0 0 0 0 0 0 0 0 0 0 0 0 0 0 0 0 0 0 0 0 0 0 0 0 0 0 0 0 0 0 0 0 0 0 0 0 0 0 0 0 0 0 0 0 0 0 0 0]  PacketSize=1400  DataTypes={'1400*uint8'}  ShowReady=off  ShowError=off  PacketID=1  ByteOrder=2  InitialValue=[]  FinalValue=[]
      settings: AttributesFormatString=TCP Protocol [27000]
  wires:
  Data Store Read1/1 -> Packet Output/1

== system PC_CONTROL_STATION/HARDWARE/RT_MONITORING/TCP 117/MSG_RX ==
  Bus Assignment : BusAssignment  AssignedSignals=RX_BUFFER
  Data Store Read : DataStoreRead  DataStoreName=MSG  IndexOptions=Index vector (dialog)  Indices=1  OutputSizes=1
  Data Store Write1 : DataStoreWrite  DataStoreName=MSG  IndexOptions=Index vector (dialog)  Indices=1  OutputSizes=1
  Packet Input : sldrtlib/Packet Input  SampleTime=CONTROL_INI.PARAM.COMM_SAMPLING_TIME  MaxMissedTicks=50  ShowMissedTicks=off  YieldWhenWaiting=off  DrvName=Standard_Devices/TCP_Protocol  DrvAddress=27001  DrvOptions=[0 27000 49 57 50 46 49 54 56 46 48 46 49 49 55 0 0 0 0 0 0 0 0 0 0 0 0 0 0 0 0 0 0 0 0 0 0 0 0 0 0 0 0 0 0 0 0 0 0 0 0 0 0 0 0 0 0 0 0 0 0 0 0 0 0 0 0 0 0 0 0 0 0 0 0 0 0 0 0 0 0 0 0 0 0 0 0 0 0 0 0 0 0 0 0 0 0 0 0 0 0 0 0 0 0 0 0 0 0 0 0 0 0 0 0 0 0 0 0 0 0 0 0 0 0 0 0 0 0 0 0 0 0 0 0 0 0 0 0 0 0 0 0 0 0 0 0 0 0 0 0 0 0 0 0 0 0 0 0 0 0 0 0 0 0 0 0 0 0 0 0 0 0 0 0 0 0 0 0 0 0 0 0 0 0 0 0 0 0 0 0 0 0 0 0 0 0 0 0 0 0 0 0 0 0 0 0 0 0 0 0 0 0 0 0 0 0 0 0 0 0 0 0 0 0 0 0 0 0 0 0 0 0 0 0 0 0 0 0 0 0 0 0 0 0 0 0 0 0 0 0 0 0 0 0 0]  PacketSize=1400  DataTypes={'1400*uint8'}  ShowReady=off  ShowError=off  PacketID=1  ByteOrder=2  ShowTimestamp=off
      settings: AttributesFormatString=TCP Protocol [27001]
  wires:
  Bus Assignment/1 -> Data Store Write1/1
  Data Store Read/1 -> Bus Assignment/1
  Packet Input/1 -> Bus Assignment/2

== system PC_CONTROL_STATION/HARDWARE/RT_MONITORING/TCP 117/MSG_TX  ==
  Enable : EnablePort
  Data Store Read1 : DataStoreRead  DataStoreName=MSG  SampleTime=CONTROL_INI.PARAM.COMM_SAMPLING_TIME  DataStoreElements=MSG.TX_BUFFER(:,1)  IndexOptions=Index vector (dialog)  Indices=1  OutputSizes=1
  Packet Output : sldrtlib/Packet Output  SampleTime=CONTROL_INI.PARAM.COMM_SAMPLING_TIME  MaxMissedTicks=50  ShowMissedTicks=off  YieldWhenWaiting=off  DrvName=Standard_Devices/TCP_Protocol  DrvAddress=27000  DrvOptions=[0 27001 49 57 50 46 49 54 56 46 48 46 49 49 55 0 0 0 0 0 0 0 0 0 0 0 0 0 0 0 0 0 0 0 0 0 0 0 0 0 0 0 0 0 0 0 0 0 0 0 0 0 0 0 0 0 0 0 0 0 0 0 0 0 0 0 0 0 0 0 0 0 0 0 0 0 0 0 0 0 0 0 0 0 0 0 0 0 0 0 0 0 0 0 0 0 0 0 0 0 0 0 0 0 0 0 0 0 0 0 0 0 0 0 0 0 0 0 0 0 0 0 0 0 0 0 0 0 0 0 0 0 0 0 0 0 0 0 0 0 0 0 0 0 0 0 0 0 0 0 0 0 0 0 0 0 0 0 0 0 0 0 0 0 0 0 0 0 0 0 0 0 0 0 0 0 0 0 0 0 0 0 0 0 0 0 0 0 0 0 0 0 0 0 0 0 0 0 0 0 0 0 0 0 0 0 0 0 0 0 0 0 0 0 0 0 0 0 0 0 0 0 0 0 0 0 0 0 0 0 0 0 0 0 0 0 0 0 0 0 0 0 0 0 0 0 0 0 0 0 0 0 0 0 0 0]  PacketSize=1400  DataTypes={'1400*uint8'}  ShowReady=off  ShowError=off  PacketID=1  ByteOrder=2  InitialValue=[]  FinalValue=[]
      settings: AttributesFormatString=TCP Protocol [27000]
  wires:
  Data Store Read1/1 -> Packet Output/1

== system PC_CONTROL_STATION/HARDWARE/RT_MONITORING/TCP 118/MSG_RX ==
  Bus Assignment : BusAssignment  AssignedSignals=RX_BUFFER
  Data Store Read : DataStoreRead  DataStoreName=MSG  IndexOptions=Index vector (dialog)  Indices=1  OutputSizes=1
  Data Store Write1 : DataStoreWrite  DataStoreName=MSG  IndexOptions=Index vector (dialog)  Indices=1  OutputSizes=1
  Packet Input : sldrtlib/Packet Input  SampleTime=SAMPLING_TIME  MaxMissedTicks=50  ShowMissedTicks=off  YieldWhenWaiting=off  DrvName=Standard_Devices/TCP_Protocol  DrvAddress=27001  DrvOptions=[0 27000 49 57 50 46 49 54 56 46 48 46 49 49 56 0 0 0 0 0 0 0 0 0 0 0 0 0 0 0 0 0 0 0 0 0 0 0 0 0 0 0 0 0 0 0 0 0 0 0 0 0 0 0 0 0 0 0 0 0 0 0 0 0 0 0 0 0 0 0 0 0 0 0 0 0 0 0 0 0 0 0 0 0 0 0 0 0 0 0 0 0 0 0 0 0 0 0 0 0 0 0 0 0 0 0 0 0 0 0 0 0 0 0 0 0 0 0 0 0 0 0 0 0 0 0 0 0 0 0 0 0 0 0 0 0 0 0 0 0 0 0 0 0 0 0 0 0 0 0 0 0 0 0 0 0 0 0 0 0 0 0 0 0 0 0 0 0 0 0 0 0 0 0 0 0 0 0 0 0 0 0 0 0 0 0 0 0 0 0 0 0 0 0 0 0 0 0 0 0 0 0 0 0 0 0 0 0 0 0 0 0 0 0 0 0 0 0 0 0 0 0 0 0 0 0 0 0 0 0 0 0 0 0 0 0 0 0 0 0 0 0 0 0 0 0 0 0 0 0 0 0 0 0 0 0]  PacketSize=1400  DataTypes={'1400*uint8'}  ShowReady=off  ShowError=off  PacketID=1  ByteOrder=2  ShowTimestamp=off
      settings: AttributesFormatString=TCP Protocol [27001]
  wires:
  Bus Assignment/1 -> Data Store Write1/1
  Data Store Read/1 -> Bus Assignment/1
  Packet Input/1 -> Bus Assignment/2

== system PC_CONTROL_STATION/HARDWARE/RT_MONITORING/TCP 118/MSG_TX  ==
  Enable : EnablePort
  Data Store Read1 : DataStoreRead  DataStoreName=MSG  SampleTime=CONTROL_INI.PARAM.COMM_SAMPLING_TIME  DataStoreElements=MSG.TX_BUFFER(:,1)  IndexOptions=Index vector (dialog)  Indices=1  OutputSizes=1
  Packet Output : sldrtlib/Packet Output  SampleTime=CONTROL_INI.PARAM.COMM_SAMPLING_TIME  MaxMissedTicks=50  ShowMissedTicks=off  YieldWhenWaiting=off  DrvName=Standard_Devices/TCP_Protocol  DrvAddress=27000  DrvOptions=[0 27001 49 57 50 46 49 54 56 46 48 46 49 49 56 0 0 0 0 0 0 0 0 0 0 0 0 0 0 0 0 0 0 0 0 0 0 0 0 0 0 0 0 0 0 0 0 0 0 0 0 0 0 0 0 0 0 0 0 0 0 0 0 0 0 0 0 0 0 0 0 0 0 0 0 0 0 0 0 0 0 0 0 0 0 0 0 0 0 0 0 0 0 0 0 0 0 0 0 0 0 0 0 0 0 0 0 0 0 0 0 0 0 0 0 0 0 0 0 0 0 0 0 0 0 0 0 0 0 0 0 0 0 0 0 0 0 0 0 0 0 0 0 0 0 0 0 0 0 0 0 0 0 0 0 0 0 0 0 0 0 0 0 0 0 0 0 0 0 0 0 0 0 0 0 0 0 0 0 0 0 0 0 0 0 0 0 0 0 0 0 0 0 0 0 0 0 0 0 0 0 0 0 0 0 0 0 0 0 0 0 0 0 0 0 0 0 0 0 0 0 0 0 0 0 0 0 0 0 0 0 0 0 0 0 0 0 0 0 0 0 0 0 0 0 0 0 0 0 0 0 0 0 0 0 0]  PacketSize=1400  DataTypes={'1400*uint8'}  ShowReady=off  ShowError=off  PacketID=1  ByteOrder=2  InitialValue=[]  FinalValue=[]
      settings: AttributesFormatString=TCP Protocol [27000]
  wires:
  Data Store Read1/1 -> Packet Output/1

== system PC_CONTROL_STATION/HARDWARE/RT_MONITORING/TCP 119/MSG_RX ==
  Bus Assignment : BusAssignment  AssignedSignals=RX_BUFFER
  Data Store Read : DataStoreRead  DataStoreName=MSG  IndexOptions=Index vector (dialog)  Indices=1  OutputSizes=1
  Data Store Write1 : DataStoreWrite  DataStoreName=MSG  IndexOptions=Index vector (dialog)  Indices=1  OutputSizes=1
  Packet Input : sldrtlib/Packet Input  SampleTime=CONTROL_INI.PARAM.COMM_SAMPLING_TIME  MaxMissedTicks=50  ShowMissedTicks=off  YieldWhenWaiting=off  DrvName=Standard_Devices/TCP_Protocol  DrvAddress=27001  DrvOptions=[0 27000 49 57 50 46 49 54 56 46 48 46 49 49 57 0 0 0 0 0 0 0 0 0 0 0 0 0 0 0 0 0 0 0 0 0 0 0 0 0 0 0 0 0 0 0 0 0 0 0 0 0 0 0 0 0 0 0 0 0 0 0 0 0 0 0 0 0 0 0 0 0 0 0 0 0 0 0 0 0 0 0 0 0 0 0 0 0 0 0 0 0 0 0 0 0 0 0 0 0 0 0 0 0 0 0 0 0 0 0 0 0 0 0 0 0 0 0 0 0 0 0 0 0 0 0 0 0 0 0 0 0 0 0 0 0 0 0 0 0 0 0 0 0 0 0 0 0 0 0 0 0 0 0 0 0 0 0 0 0 0 0 0 0 0 0 0 0 0 0 0 0 0 0 0 0 0 0 0 0 0 0 0 0 0 0 0 0 0 0 0 0 0 0 0 0 0 0 0 0 0 0 0 0 0 0 0 0 0 0 0 0 0 0 0 0 0 0 0 0 0 0 0 0 0 0 0 0 0 0 0 0 0 0 0 0 0 0 0 0 0 0 0 0 0 0 0 0 0 0 0 0 0 0 0 0]  PacketSize=1400  DataTypes={'1400*uint8'}  ShowReady=off  ShowError=off  PacketID=1  ByteOrder=2  ShowTimestamp=off
      settings: AttributesFormatString=TCP Protocol [27001]
  wires:
  Bus Assignment/1 -> Data Store Write1/1
  Data Store Read/1 -> Bus Assignment/1
  Packet Input/1 -> Bus Assignment/2

== system PC_CONTROL_STATION/HARDWARE/RT_MONITORING/TCP 119/MSG_TX  ==
  Enable : EnablePort
  Data Store Read1 : DataStoreRead  DataStoreName=MSG  SampleTime=CONTROL_INI.PARAM.COMM_SAMPLING_TIME  DataStoreElements=MSG.TX_BUFFER(:,1)  IndexOptions=Index vector (dialog)  Indices=1  OutputSizes=1
  Packet Output : sldrtlib/Packet Output  SampleTime=CONTROL_INI.PARAM.COMM_SAMPLING_TIME  MaxMissedTicks=50  ShowMissedTicks=off  YieldWhenWaiting=off  DrvName=Standard_Devices/TCP_Protocol  DrvAddress=27000  DrvOptions=[0 27001 49 57 50 46 49 54 56 46 48 46 49 49 57 0 0 0 0 0 0 0 0 0 0 0 0 0 0 0 0 0 0 0 0 0 0 0 0 0 0 0 0 0 0 0 0 0 0 0 0 0 0 0 0 0 0 0 0 0 0 0 0 0 0 0 0 0 0 0 0 0 0 0 0 0 0 0 0 0 0 0 0 0 0 0 0 0 0 0 0 0 0 0 0 0 0 0 0 0 0 0 0 0 0 0 0 0 0 0 0 0 0 0 0 0 0 0 0 0 0 0 0 0 0 0 0 0 0 0 0 0 0 0 0 0 0 0 0 0 0 0 0 0 0 0 0 0 0 0 0 0 0 0 0 0 0 0 0 0 0 0 0 0 0 0 0 0 0 0 0 0 0 0 0 0 0 0 0 0 0 0 0 0 0 0 0 0 0 0 0 0 0 0 0 0 0 0 0 0 0 0 0 0 0 0 0 0 0 0 0 0 0 0 0 0 0 0 0 0 0 0 0 0 0 0 0 0 0 0 0 0 0 0 0 0 0 0 0 0 0 0 0 0 0 0 0 0 0 0 0 0 0 0 0 0]  PacketSize=1400  DataTypes={'1400*uint8'}  ShowReady=off  ShowError=off  PacketID=1  ByteOrder=2  InitialValue=[]  FinalValue=[]
      settings: AttributesFormatString=TCP Protocol [27000]
  wires:
  Data Store Read1/1 -> Packet Output/1

== system PC_CONTROL_STATION/HARDWARE/RT_MONITORING/TCP 120/MSG_RX ==
  Bus Assignment : BusAssignment  AssignedSignals=RX_BUFFER
  Data Store Read : DataStoreRead  DataStoreName=MSG  IndexOptions=Index vector (dialog)  Indices=1  OutputSizes=1
  Data Store Write1 : DataStoreWrite  DataStoreName=MSG  IndexOptions=Index vector (dialog)  Indices=1  OutputSizes=1
  Packet Input : sldrtlib/Packet Input  SampleTime=CONTROL_INI.PARAM.COMM_SAMPLING_TIME  MaxMissedTicks=50  ShowMissedTicks=off  YieldWhenWaiting=off  DrvName=Standard_Devices/TCP_Protocol  DrvAddress=27001  DrvOptions=[0 27000 49 57 50 46 49 54 56 46 49 46 49 57 0 0 0 0 0 0 0 0 0 0 0 0 0 0 0 0 0 0 0 0 0 0 0 0 0 0 0 0 0 0 0 0 0 0 0 0 0 0 0 0 0 0 0 0 0 0 0 0 0 0 0 0 0 0 0 0 0 0 0 0 0 0 0 0 0 0 0 0 0 0 0 0 0 0 0 0 0 0 0 0 0 0 0 0 0 0 0 0 0 0 0 0 0 0 0 0 0 0 0 0 0 0 0 0 0 0 0 0 0 0 0 0 0 0 0 0 0 0 0 0 0 0 0 0 0 0 0 0 0 0 0 0 0 0 0 0 0 0 0 0 0 0 0 0 0 0 0 0 0 0 0 0 0 0 0 0 0 0 0 0 0 0 0 0 0 0 0 0 0 0 0 0 0 0 0 0 0 0 0 0 0 0 0 0 0 0 0 0 0 0 0 0 0 0 0 0 0 0 0 0 0 0 0 0 0 0 0 0 0 0 0 0 0 0 0 0 0 0 0 0 0 0 0 0 0 0 0 0 0 0 0 0 0 0 0 0 0 0 0 0 0 0]  PacketSize=1400  DataTypes={'1400*uint8'}  ShowReady=off  ShowError=off  PacketID=1  ByteOrder=2  ShowTimestamp=off
      settings: AttributesFormatString=TCP Protocol [27001]
  wires:
  Bus Assignment/1 -> Data Store Write1/1
  Data Store Read/1 -> Bus Assignment/1
  Packet Input/1 -> Bus Assignment/2

== system PC_CONTROL_STATION/HARDWARE/RT_MONITORING/TCP 120/MSG_TX  ==
  Enable : EnablePort
  Data Store Read1 : DataStoreRead  DataStoreName=MSG  SampleTime=CONTROL_INI.PARAM.COMM_SAMPLING_TIME  DataStoreElements=MSG.TX_BUFFER(:,1)  IndexOptions=Index vector (dialog)  Indices=1  OutputSizes=1
  Packet Output : sldrtlib/Packet Output  SampleTime=CONTROL_INI.PARAM.COMM_SAMPLING_TIME  MaxMissedTicks=50  ShowMissedTicks=off  YieldWhenWaiting=off  DrvName=Standard_Devices/TCP_Protocol  DrvAddress=27000  DrvOptions=[0 27001 49 57 50 46 49 54 56 46 49 46 49 57 0 0 0 0 0 0 0 0 0 0 0 0 0 0 0 0 0 0 0 0 0 0 0 0 0 0 0 0 0 0 0 0 0 0 0 0 0 0 0 0 0 0 0 0 0 0 0 0 0 0 0 0 0 0 0 0 0 0 0 0 0 0 0 0 0 0 0 0 0 0 0 0 0 0 0 0 0 0 0 0 0 0 0 0 0 0 0 0 0 0 0 0 0 0 0 0 0 0 0 0 0 0 0 0 0 0 0 0 0 0 0 0 0 0 0 0 0 0 0 0 0 0 0 0 0 0 0 0 0 0 0 0 0 0 0 0 0 0 0 0 0 0 0 0 0 0 0 0 0 0 0 0 0 0 0 0 0 0 0 0 0 0 0 0 0 0 0 0 0 0 0 0 0 0 0 0 0 0 0 0 0 0 0 0 0 0 0 0 0 0 0 0 0 0 0 0 0 0 0 0 0 0 0 0 0 0 0 0 0 0 0 0 0 0 0 0 0 0 0 0 0 0 0 0 0 0 0 0 0 0 0 0 0 0 0 0 0 0 0 0 0 0]  PacketSize=1400  DataTypes={'1400*uint8'}  ShowReady=off  ShowError=off  PacketID=1  ByteOrder=2  InitialValue=[]  FinalValue=[]
      settings: AttributesFormatString=TCP Protocol [27000]
  wires:
  Data Store Read1/1 -> Packet Output/1

== system PC_CONTROL_STATION/HARDWARE/RT_MONITORING/TCP 121/MSG_RX ==
  Bus Assignment : BusAssignment  AssignedSignals=RX_BUFFER
  Data Store Read : DataStoreRead  DataStoreName=MSG  IndexOptions=Index vector (dialog)  Indices=1  OutputSizes=1
  Data Store Write1 : DataStoreWrite  DataStoreName=MSG  IndexOptions=Index vector (dialog)  Indices=1  OutputSizes=1
  Packet Input : sldrtlib/Packet Input  SampleTime=CONTROL_INI.PARAM.COMM_SAMPLING_TIME  MaxMissedTicks=50  ShowMissedTicks=off  YieldWhenWaiting=off  DrvName=Standard_Devices/TCP_Protocol  DrvAddress=27001  DrvOptions=[0 27000 49 57 50 46 49 54 56 46 48 46 49 50 49 0 0 0 0 0 0 0 0 0 0 0 0 0 0 0 0 0 0 0 0 0 0 0 0 0 0 0 0 0 0 0 0 0 0 0 0 0 0 0 0 0 0 0 0 0 0 0 0 0 0 0 0 0 0 0 0 0 0 0 0 0 0 0 0 0 0 0 0 0 0 0 0 0 0 0 0 0 0 0 0 0 0 0 0 0 0 0 0 0 0 0 0 0 0 0 0 0 0 0 0 0 0 0 0 0 0 0 0 0 0 0 0 0 0 0 0 0 0 0 0 0 0 0 0 0 0 0 0 0 0 0 0 0 0 0 0 0 0 0 0 0 0 0 0 0 0 0 0 0 0 0 0 0 0 0 0 0 0 0 0 0 0 0 0 0 0 0 0 0 0 0 0 0 0 0 0 0 0 0 0 0 0 0 0 0 0 0 0 0 0 0 0 0 0 0 0 0 0 0 0 0 0 0 0 0 0 0 0 0 0 0 0 0 0 0 0 0 0 0 0 0 0 0 0 0 0 0 0 0 0 0 0 0 0 0 0 0 0 0 0 0]  PacketSize=1400  DataTypes={'1400*uint8'}  ShowReady=off  ShowError=off  PacketID=1  ByteOrder=2  ShowTimestamp=off
      settings: AttributesFormatString=TCP Protocol [27001]
  wires:
  Bus Assignment/1 -> Data Store Write1/1
  Data Store Read/1 -> Bus Assignment/1
  Packet Input/1 -> Bus Assignment/2

== system PC_CONTROL_STATION/HARDWARE/RT_MONITORING/TCP 121/MSG_TX  ==
  Enable : EnablePort
  Data Store Read1 : DataStoreRead  DataStoreName=MSG  SampleTime=CONTROL_INI.PARAM.COMM_SAMPLING_TIME  DataStoreElements=MSG.TX_BUFFER(:,1)  IndexOptions=Index vector (dialog)  Indices=1  OutputSizes=1
  Packet Output : sldrtlib/Packet Output  SampleTime=CONTROL_INI.PARAM.COMM_SAMPLING_TIME  MaxMissedTicks=50  ShowMissedTicks=off  YieldWhenWaiting=off  DrvName=Standard_Devices/TCP_Protocol  DrvAddress=27000  DrvOptions=[0 27001 49 57 50 46 49 54 56 46 48 46 49 50 49 0 0 0 0 0 0 0 0 0 0 0 0 0 0 0 0 0 0 0 0 0 0 0 0 0 0 0 0 0 0 0 0 0 0 0 0 0 0 0 0 0 0 0 0 0 0 0 0 0 0 0 0 0 0 0 0 0 0 0 0 0 0 0 0 0 0 0 0 0 0 0 0 0 0 0 0 0 0 0 0 0 0 0 0 0 0 0 0 0 0 0 0 0 0 0 0 0 0 0 0 0 0 0 0 0 0 0 0 0 0 0 0 0 0 0 0 0 0 0 0 0 0 0 0 0 0 0 0 0 0 0 0 0 0 0 0 0 0 0 0 0 0 0 0 0 0 0 0 0 0 0 0 0 0 0 0 0 0 0 0 0 0 0 0 0 0 0 0 0 0 0 0 0 0 0 0 0 0 0 0 0 0 0 0 0 0 0 0 0 0 0 0 0 0 0 0 0 0 0 0 0 0 0 0 0 0 0 0 0 0 0 0 0 0 0 0 0 0 0 0 0 0 0 0 0 0 0 0 0 0 0 0 0 0 0 0 0 0 0 0 0]  PacketSize=1400  DataTypes={'1400*uint8'}  ShowReady=off  ShowError=off  PacketID=1  ByteOrder=2  InitialValue=[]  FinalValue=[]
      settings: AttributesFormatString=TCP Protocol [27000]
  wires:
  Data Store Read1/1 -> Packet Output/1

== system PC_CONTROL_STATION/HARDWARE/RT_MONITORING/TCP RSP/MSG_RX ==
  Bus Assignment : BusAssignment  AssignedSignals=RX_BUFFER
  Data Store Read : DataStoreRead  DataStoreName=MSG  IndexOptions=Index vector (dialog)  Indices=1  OutputSizes=1
  Data Store Write1 : DataStoreWrite  DataStoreName=MSG  IndexOptions=Index vector (dialog)  Indices=1  OutputSizes=1
  Packet Input : sldrtlib/Packet Input  SampleTime=CONTROL_INI.PARAM.COMM_SAMPLING_TIME  MaxMissedTicks=50  ShowMissedTicks=off  YieldWhenWaiting=off  DrvName=Standard_Devices/TCP_Protocol  DrvAddress=27001  DrvOptions=[0 27000 49 57 50 46 49 54 56 46 48 46 50 51 52 0 0 0 0 0 0 0 0 0 0 0 0 0 0 0 0 0 0 0 0 0 0 0 0 0 0 0 0 0 0 0 0 0 0 0 0 0 0 0 0 0 0 0 0 0 0 0 0 0 0 0 0 0 0 0 0 0 0 0 0 0 0 0 0 0 0 0 0 0 0 0 0 0 0 0 0 0 0 0 0 0 0 0 0 0 0 0 0 0 0 0 0 0 0 0 0 0 0 0 0 0 0 0 0 0 0 0 0 0 0 0 0 0 0 0 0 0 0 0 0 0 0 0 0 0 0 0 0 0 0 0 0 0 0 0 0 0 0 0 0 0 0 0 0 0 0 0 0 0 0 0 0 0 0 0 0 0 0 0 0 0 0 0 0 0 0 0 0 0 0 0 0 0 0 0 0 0 0 0 0 0 0 0 0 0 0 0 0 0 0 0 0 0 0 0 0 0 0 0 0 0 0 0 0 0 0 0 0 0 0 0 0 0 0 0 0 0 0 0 0 0 0 0 0 0 0 0 0 0 0 0 0 0 0 0 0 0 0 0 0 0]  PacketSize=1400  DataTypes={'1400*uint8'}  ShowReady=off  ShowError=off  PacketID=1  ByteOrder=2  ShowTimestamp=off
      settings: AttributesFormatString=TCP Protocol [27001]
  wires:
  Bus Assignment/1 -> Data Store Write1/1
  Data Store Read/1 -> Bus Assignment/1
  Packet Input/1 -> Bus Assignment/2

== system PC_CONTROL_STATION/HARDWARE/RT_MONITORING/TCP RSP/MSG_TX  ==
  Enable : EnablePort
  Data Store Read1 : DataStoreRead  DataStoreName=MSG  SampleTime=CONTROL_INI.PARAM.COMM_SAMPLING_TIME  DataStoreElements=MSG.TX_BUFFER(:,1)  IndexOptions=Index vector (dialog)  Indices=1  OutputSizes=1
  Packet Output : sldrtlib/Packet Output  SampleTime=CONTROL_INI.PARAM.COMM_SAMPLING_TIME  MaxMissedTicks=50  ShowMissedTicks=off  YieldWhenWaiting=off  DrvName=Standard_Devices/TCP_Protocol  DrvAddress=27000  DrvOptions=[0 27001 49 57 50 46 49 54 56 46 48 46 50 51 52 0 0 0 0 0 0 0 0 0 0 0 0 0 0 0 0 0 0 0 0 0 0 0 0 0 0 0 0 0 0 0 0 0 0 0 0 0 0 0 0 0 0 0 0 0 0 0 0 0 0 0 0 0 0 0 0 0 0 0 0 0 0 0 0 0 0 0 0 0 0 0 0 0 0 0 0 0 0 0 0 0 0 0 0 0 0 0 0 0 0 0 0 0 0 0 0 0 0 0 0 0 0 0 0 0 0 0 0 0 0 0 0 0 0 0 0 0 0 0 0 0 0 0 0 0 0 0 0 0 0 0 0 0 0 0 0 0 0 0 0 0 0 0 0 0 0 0 0 0 0 0 0 0 0 0 0 0 0 0 0 0 0 0 0 0 0 0 0 0 0 0 0 0 0 0 0 0 0 0 0 0 0 0 0 0 0 0 0 0 0 0 0 0 0 0 0 0 0 0 0 0 0 0 0 0 0 0 0 0 0 0 0 0 0 0 0 0 0 0 0 0 0 0 0 0 0 0 0 0 0 0 0 0 0 0 0 0 0 0 0 0]  PacketSize=1400  DataTypes={'1400*uint8'}  ShowReady=off  ShowError=off  PacketID=1  ByteOrder=2  InitialValue=[]  FinalValue=[]
      settings: AttributesFormatString=TCP Protocol [27000]
  wires:
  Data Store Read1/1 -> Packet Output/1

== system PC_CONTROL_STATION/HARDWARE/RT_MONITORING/UDP/MSG_RX ==
  Bus Assignment : BusAssignment  AssignedSignals=RX_BUFFER
  Data Store Read : DataStoreRead  DataStoreName=MSG  IndexOptions=Index vector (dialog)  Indices=1  OutputSizes=1
  Data Store Write1 : DataStoreWrite  DataStoreName=MSG  IndexOptions=Index vector (dialog)  Indices=1  OutputSizes=1
  Display : Display
  Packet Input : sldrtlib/Packet Input  SampleTime=CONTROL_INI.PARAM.COMM_SAMPLING_TIME  MaxMissedTicks=50  ShowMissedTicks=off  YieldWhenWaiting=off  DrvName=Standard_Devices/UDP_Protocol  DrvAddress=37000  DrvOptions=[0 37001 49 57 50 46 49 54 56 46 49 46 51 56 0 0 0 0 0 0 0 0 0 0 0 0 0 0 0 0 0 0 0 0 0 0 0 0 0 0 0 0 0 0 0 0 0 0 0 0 0 0 0 0 0 0 0 0 0 0 0 0 0 0 0 0 0 0 0 0 0 0 0 0 0 0 0 0 0 0 0 0 0 0 0 0 0 0 0 0 0 0 0 0 0 0 0 0 0 0 0 0 0 0 0 0 0 0 0 0 0 0 0 0 0 0 0 0 0 0 0 0 0 0 0 0 0 0 0 0 0 0 0 0 0 0 0 0 0 0 0 0 0 0 0 0 0 0 0 0 0 0 0 0 0 0 0 0 0 0 0 0 0 0 0 0 0 0 0 0 0 0 0 0 0 0 0 0 0 0 0 0 0 0 0 0 0 0 0 0 0 0 0 0 0 0 0 0 0 0 0 0 0 0 0 0 0 0 0 0 0 0 0 0 0 0 0 0 0 0 0 0 0 0 0 0 0 0 0 0 0 0 0 0 0 0 0 0 0 0 0 0 0 0 0 0 0 0 0 0 0 0 0 0 0 0]  PacketSize=255  DataTypes={'255*uint8'}  ShowReady=off  ShowError=off  PacketID=1  ByteOrder=1  ShowTimestamp=off
      settings: AttributesFormatString=UDP Protocol [37000]
  wires:
  Bus Assignment/1 -> Data Store Write1/1
  Data Store Read/1 -> Bus Assignment/1
  Packet Input/1 -> Bus Assignment/2, Display/1

== system PC_CONTROL_STATION/HARDWARE/RT_MONITORING/UDP/MSG_TX  ==
  Enable : EnablePort
  Data Store Read1 : DataStoreRead  DataStoreName=MSG  SampleTime=CONTROL_INI.PARAM.COMM_SAMPLING_TIME  DataStoreElements=MSG.TX_BUFFER(:,1)  IndexOptions=Index vector (dialog)  Indices=1  OutputSizes=1
  Display : Display
  Packet Output : sldrtlib/Packet Output  SampleTime=CONTROL_INI.PARAM.COMM_SAMPLING_TIME  MaxMissedTicks=50  ShowMissedTicks=off  YieldWhenWaiting=off  DrvName=Standard_Devices/UDP_Protocol  DrvAddress=37000  DrvOptions=[0 37001 49 57 50 46 49 54 56 46 49 46 51 56 0 0 0 0 0 0 0 0 0 0 0 0 0 0 0 0 0 0 0 0 0 0 0 0 0 0 0 0 0 0 0 0 0 0 0 0 0 0 0 0 0 0 0 0 0 0 0 0 0 0 0 0 0 0 0 0 0 0 0 0 0 0 0 0 0 0 0 0 0 0 0 0 0 0 0 0 0 0 0 0 0 0 0 0 0 0 0 0 0 0 0 0 0 0 0 0 0 0 0 0 0 0 0 0 0 0 0 0 0 0 0 0 0 0 0 0 0 0 0 0 0 0 0 0 0 0 0 0 0 0 0 0 0 0 0 0 0 0 0 0 0 0 0 0 0 0 0 0 0 0 0 0 0 0 0 0 0 0 0 0 0 0 0 0 0 0 0 0 0 0 0 0 0 0 0 0 0 0 0 0 0 0 0 0 0 0 0 0 0 0 0 0 0 0 0 0 0 0 0 0 0 0 0 0 0 0 0 0 0 0 0 0 0 0 0 0 0 0 0 0 0 0 0 0 0 0 0 0 0 0 0 0 0 0 0 0 0 0 0 0 0 0]  PacketSize=255  DataTypes={'255*uint8'}  ShowReady=off  ShowError=off  PacketID=1  ByteOrder=1  InitialValue=[]  FinalValue=[]
      settings: AttributesFormatString=UDP Protocol [37000]
  wires:
  Data Store Read1/1 -> Packet Output/1, Display/1

== matlab function PC_CONTROL_STATION/PC TARGETS/PC TARGETS/FORWARD VELOCITY TARGET/ PULSE GENERATION ==
  data: CONTROL input Bus: CONTROL_Bus; FORWARD_VEL_REF output
function FORWARD_VEL_REF = PULSE_GEN(CONTROL)
    
persistent TIMER initialize
if isempty(initialize)
    TIMER = 0;
    initialize = 1;
end

% SAMPLING TIME
SAMPLING_TIME = CONTROL.PARAM.SAMPLING_TIME; % s

%% OPERATION MODE
% / 0. BOOTING   / 1. SENSOR CALIBRATION / 2. READY
% / 3. OPEN LOOP / 4. ATTITUDE / 5. VELOCITY / 6. NAVIGATION / 
% / 7. WALL FOLLOWER / 8. WALL-FOLLOWER COMPETITION / 
% / 9. NAVIGATION COMPETITION / 10. STOP
CURRENT_STATUS = CONTROL.STATE.CURRENT_STATUS_SYS;
PREVIOUS_STATUS = CONTROL.STATE.PREVIOUS_STATUS;

if (CURRENT_STATUS == 5) && (PREVIOUS_STATUS == 5)   
    if TIMER > 7.5
        FORWARD_VEL_REF = 0;
    elseif TIMER < 5
        FORWARD_VEL_REF = 0;
        TIMER = TIMER + SAMPLING_TIME;
    else % 5 <= TIMER <= 7.5
        FORWARD_VEL_REF = 0.25;
        TIMER = TIMER + SAMPLING_TIME;
    end
else
    FORWARD_VEL_REF = 0;
    TIMER = 0;
end
